simulink model "arm_angle_pid"  (R2022b)
settings: Solver=FixedStepDiscrete  StartTime=0.0  StopTime=inf  RelTol=1e-3
undefined symbols (not defined in the file or in its folder): deltaT
libraries: arduinolib x4, slpidlib x1, simulink x1
settings Model: SimulationMode=external  ExtModeTrigDuration=2  Creator=alpdemir  LastModifiedBy=Volkan
settings SolverCC: AlgebraicLoopSolver=TrustRegion
settings DataIOCC: LimitDataPoints=on  MaxDataPoints=5000  InspectSignalLogs=on  ReturnWorkspaceOutputs=off
settings OptimizationCC: MaxStackSize=64  EfficientTunableParamExpr=on
settings DebuggingCC: ParameterTunabilityLossMsg=error  UnconnectedInputMsg=warning  UnconnectedOutputMsg=warning  UnconnectedLineMsg=warning  SFMachineParentedDataDiag=warning  ArithmeticOperatorsInVariantConditions=warning
settings HardwareCC: ProdBitPerInt=16  ProdBitPerPointer=16  ProdBitPerSizeT=16  ProdBitPerPtrDiffT=16  ProdLargestAtomicFloat=None  ProdWordSize=8  ProdHWDeviceType=Atmel->AVR
settings ModelReferenceCC: EnableRefExpFcnMdlSchedulingChecks=on
settings SFSimCC: SimUseLocalCustomCode=off  MATLABDynamicMemAlloc=off  CustomCodeUndefinedFunction=UseInterfaceOnly
settings RTWCC: Description=Embedded Coder  SystemTargetFile=ert.tlc  HardwareBoard=Arduino Uno  TLCOptions=-aInlineSetEventsForThisBaseRateFcn=TLC_FALSE -aSuppressMultiTaskScheduler=TLC_FALSE -aRateBasedStepFcn=1  TemplateMakefile=ert_default_tmf  GenerateReport=on  RTWUseLocalCustomCode=off  Toolchain=Arduino AVR  BuildConfiguration=Faster Runs  IncludeHyperlinkInReport=on  LaunchReport=on  GenerateTraceInfo=on  GenerateTraceReport=on  GenerateTraceReportSl=on  GenerateTraceReportSf=on  GenerateTraceReportEml=on
settings CodeAppCC: ForceParamTrailComments=on  IgnoreCustomStorageClasses=off  OperatorAnnotations=on  SimulinkDataObjDesc=on  SFDataObjDesc=on  MATLABFcnDesc=on  InsertBlockDesc=on  StateflowObjectComments=on  MATLABSourceComments=on
settings ERTTargetCC: MultiwordLength=2048  SupportContinuousTime=on  SupportVariableSizeSignals=on

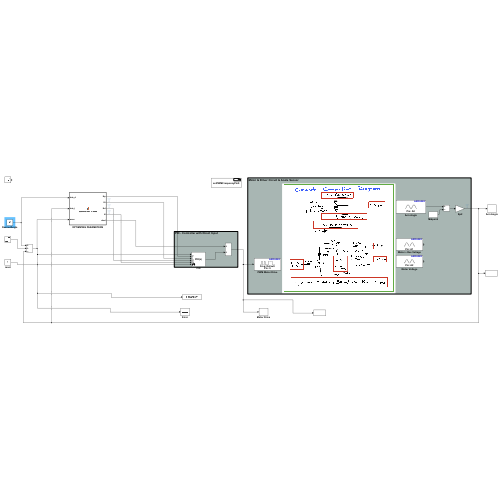
[thumbnail: Simulink's stored preview of the top-level diagram]
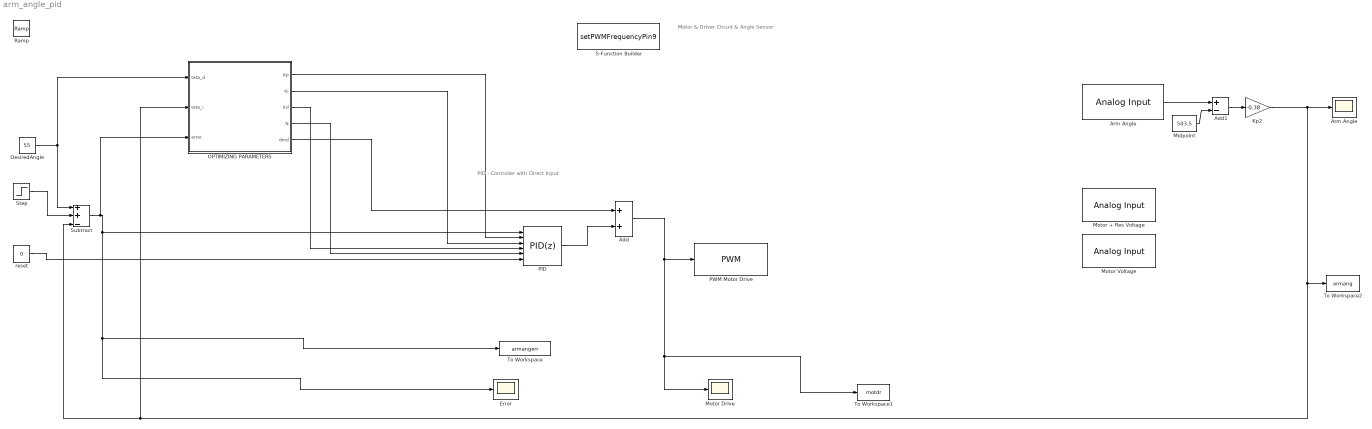
== system arm_angle_pid ==
  note: Motor & Driver Circuit & Angle Sensor
  note: PID - Controller with Direct Input
  Add : Sum
  Add1 : Sum  Inputs=+-
  Arm Angle : arduinolib/Analog Input  pinNumber=0  ReadResultsOnly=off  ConversionTriggerSource=Software  ExternalTriggerType=uint32( 0 )  OutputDataType=uint16  EnableConversionCompleteNotify=off  EnableOuputStatus=off  SampleTime=deltaT  blockPlatform=arduino
  "Arm Angle " : Scope
  DesiredAngle : Constant  Value=55
  Error : Scope
  Kp2 : Gain  Gain=-0.38
  Midpoint : Constant  Value=503.5
  Motor + Res Voltage : arduinolib/Analog Input  pinNumber=1  ReadResultsOnly=off  ConversionTriggerSource=Software  ExternalTriggerType=uint32( 0 )  OutputDataType=uint16  EnableConversionCompleteNotify=off  EnableOuputStatus=off  SampleTime=deltaT  blockPlatform=arduino
  Motor Drive : Scope
  Motor Voltage : arduinolib/Analog Input  pinNumber=2  ReadResultsOnly=off  ConversionTriggerSource=Software  ExternalTriggerType=uint32( 0 )  OutputDataType=uint16  EnableConversionCompleteNotify=off  EnableOuputStatus=off  SampleTime=deltaT  blockPlatform=arduino
  OPTIMIZING PARAMETERS : MATLAB Function  TreatAsAtomicUnit=on
  PID : slpidlib/PID Controller  Controller=PID  Form=Ideal  TimeDomain=Discrete-time  UseExternalTs=off  SampleTime=-1  IntegratorMethod=Forward Euler  FilterMethod=Forward Euler  ControllerParametersSource=external  P=1.1  I=0.7  UseKiTs=off  D=0.5  N=80  UseFilter=on  TunerSelectOption=Transfer Function Based (PID Tuner App)  ZeroCross=off  InitialConditionSource=internal  InitialConditionForIntegrator=0  InitialConditionForFilter=0  DifferentiatorICPrevScaledInput=0  ExternalReset=either  TrackingMode=off  Kt=1  LimitOutput=off  SatLimitsSource=internal  UpperSaturationLimit=50  LowerSaturationLimit=-50  LinearizeAsGain=off  AntiWindupMode=none  Kb=1  LimitIntegrator=off  UpperIntegratorSaturationLimit=inf  LowerIntegratorSaturationLimit=-inf  POutMin=[]  POutMax=[]  IOutMin=[]  IOutMax=[]  DOutMin=[]  DOutMax=[]  NOutMin=[]  NOutMax=[]  SumOutMin=[]  SumOutMax=[]  SaturationOutMin=[]  SaturationOutMax=[]  PParamMin=[]  PParamMax=[]  IParamMin=[]  IParamMax=[]  DParamMin=[]  DParamMax=[]  NParamMin=[]  NParamMax=[]  KbParamMin=[]  KbParamMax=[]  KtParamMin=[]  KtParamMax=[]  KbOutMin=[]  KbOutMax=[]  KtOutMin=[]  KtOutMax=[]  IntegratorOutMin=[]  IntegratorOutMax=[]  FilterOutMin=[]  FilterOutMax=[]  SumI1OutMin=[]  SumI1OutMax=[]  SumI2OutMin=[]  SumI2OutMax=[]  SumI3OutMin=[]  SumI3OutMax=[]  SumI4OutMin=[]  SumI4OutMax=[]  SumDOutMin=[]  SumDOutMax=[]  DifferentiatorOutMin=[]  DifferentiatorOutMax=[]  FilterDiffOutCoefMin=[]  FilterDiffOutCoefMax=[]  ReciprocalOutMin=[]  ReciprocalOutMax=[]  SumDenOutMin=[]  SumDenOutMax=[]  SumNumOutMin=[]  SumNumOutMax=[]  DivideOutMin=[]  DivideOutMax=[]  UdiffTsProdOutMin=[]  UdiffTsProdOutMax=[]  NTsProdOutMin=[]  NTsProdOutMax=[]  UintegralTsProdOutMin=[]  UintegralTsProdOutMax=[]  UngainTsProdOutMin=[]  UngainTsProdOutMax=[]  ClampingZeroOutDataTypeStr=Inherit: Inherit via back propagation  ClampingZeroOutMin=[]  ClampingZeroOutMax=[]  FilterDenConstantOutDataTypeStr=Inherit: Inherit via back propagation  FilterDenConstantOutMin=[]  FilterDenConstantOutMax=[]  PCopyOutDataTypeStr=Inherit: Inherit via back propagation  PCopyOutMin=[]  PCopyOutMax=[]  NCopyOutDataTypeStr=Inherit: Inherit via back propagation  NCopyOutMin=[]  NCopyOutMax=[]  IntegratorContinuousStateAttributes=''  IntegratorStateMustResolveToSignalObject=off  IntegratorRTWStateStorageClass=Auto  FilterContinuousStateAttributes=''  FilterStateMustResolveToSignalObject=off  FilterRTWStateStorageClass=Auto  ParallelPVariant=Passthrough  IdealPVariant=ExternalParameters  IVariant=ExternalParameters  DVariant=ExternalParameters  IntegratorVariant=Discrete  SatVariant=Disabled  AWVariant=Passthrough  PCopyVariant=Disabled  TRVariant=Disabled  FdbkBlocksVariant=Forward  IdealPFdbkVariant=Disabled  SatFdbkVariant=Disabled  DerivativeFilterVariant=ForwardEulerFilter  NVariant=ExternalParameters  NCopyVariant=Disabled  FilterICVariant=InternalICsFilter  IntegratorICVariant=InternalICs  ExternalResetVariant=ExternalReset  TRSumVariant=Passthrough  SumFdbkVariant=Disabled  SumVariant=Sum_PID  TsampFilterVariant=InternalTs  TsampNgainVariant=Passthrough  TsampIntegralVariant=Passthrough  ExternalSaturationOutDataTypeStr=Inherit: Same as second input
  PWM Motor Drive : arduinolib/PWM  pinNumber=9  frequencyType=Default  desiredFrequency=490.2  achievableFrequency=490.2
  Ramp : simulink/Sources/Ramp  slope=1  start=0  InitialOutput=0
  S-Function Builder : S-Function  InitFcn=try, set_param(gcb,'FunctionName','setPWMFrequencyPin9'), end  FunctionName=setPWMFrequencyPin9  SFunctionModules=setPWMFrequencyPin9_wrapper  SFunctionDeploymentMode=off  EnableBusSupport=off  mask(S-Function Builder){}
      mask help: Simulink:masks:SFunctionBuilder_MD
      mask init:
      | val = [[.9  0.75 0.75 1 1 .9 .9 1]',[1 1 0.75 0.75 .9 .9 1 .9]'];try , sys = get_param(gcb,'SfunBuilderFcnName');if isempty(sys), sys = get_param(gcb,'FunctionName'); end,catch, sys = get_param(gcb,'FunctionName'); end
      settings: CopyFcn=set_param(gcbh,'LinkStatus','none')  PreSaveFcn=try, set_param(gcb,'FunctionName','setPWMFrequencyPin9'), end  OpenFcn=sfunctionwizard(gcbh)
      mask Display:
      | plot(val(:,1),val(:,2))
      | disp(sys)
  Step : Step  Time=0  After=0  SampleTime=deltaT
  Subtract : Sum  Inputs=++-
  To Workspace : ToWorkspace  VariableName=armangerr  SaveFormat=Structure With Time  SampleTime=-1
      settings: MaxDataPoints=1000001
  To Workspace1 : ToWorkspace  VariableName=motdr  SaveFormat=Structure With Time  SampleTime=-1
      settings: MaxDataPoints=1000001
  To Workspace2 : ToWorkspace  VariableName=armang  SaveFormat=Structure With Time  SampleTime=-1
      settings: MaxDataPoints=1000001
  reset : Constant  Value=0
  wires:
  Subtract/1 -> OPTIMIZING PARAMETERS/3(error), Error/1, To Workspace/1, PID/1
  Midpoint/1 -> Add1/2
  Arm Angle/1 -> Add1/1
  Add1/1 -> Kp2/1
  Kp2/1 -> "Arm Angle "/1, To Workspace2/1, Subtract/3, OPTIMIZING PARAMETERS/2(teta_i)
  PID/1 -> Add/2
  DesiredAngle/1 -> Subtract/1, OPTIMIZING PARAMETERS/1(teta_d)
  Add/1 -> To Workspace1/1, Motor Drive/1, PWM Motor Drive/1
  Step/1 -> Subtract/2
  reset/1 -> PID/6
  OPTIMIZING PARAMETERS/5(dmd) -> Add/1
  OPTIMIZING PARAMETERS/4(N) -> PID/5
  OPTIMIZING PARAMETERS/3(Kd) -> PID/4
  OPTIMIZING PARAMETERS/2(Ki) -> PID/3
  OPTIMIZING PARAMETERS/1(Kp) -> PID/2

== matlab function arm_angle_pid/OPTIMIZING PARAMETERS ==
  data: teta_d input; Kp output; teta_i input; Ki output; Kd output; N output; dmd output; error input

function [Kp,Ki,Kd,N,dmd] = optimizeParameters(teta_d,teta_i,error)  
        dmd=0;
        if(teta_d<65 && teta_d>10)   
                Kp=1.15;
                Ki=0.15;
                Kd=0.25;
                N=90;
                dmd=-((16+error*4/135));
            
                if error>40
                    Ki=0.35;
                elseif error>30
                    Ki=0.30;
                elseif error>20
                    Ki=0.25;
                elseif error>10
                    Ki=0.20;
                else
                    Ki=0.15;
                end
              
        elseif(teta_d<10 && teta_d>-10)
            Kp=1.1;
            Ki=0.35;
            Kd=0.3;
            N=90;
            dmd=6.5*(cosd(teta_i))+4;

        elseif(teta_d>=55)   
            Kp=1.05;
            Ki=0.16;
            Kd=0.35;
            N=90;
            dmd=-(abs(45-error*8/135))-20;

        elseif teta_d<=-10
            Kp=1.1;
            Ki=0.7;
            Kd=0.5;
            N=80;
            dmd=0;

        else
            Kp=0;
            Ki=0;
            Kd=0;
            N=0;
            dmd=0;
        end
end
